simulink model "AOO"  (R2022a)
settings: Solver=FixedStepAuto  StartTime=0.0  StopTime=inf  FixedStep=1e-3  RelTol=1e-3  EnableMultiTasking=on
undefined symbols (not defined in the file): D10, D11, D12, D2, D4, D5, D7, D8, D9, PTA0, PTA2, PTB23, PTB9, PTC3, PTC4, PTD0, PTD2, PTD3
libraries: frdmk64flib x9
settings Model: ExtModeTrigDuration=5  Creator=ethan  LastModifiedBy=taimu
settings OptimizationCC: EnhancedBackFolding=on  PassReuseOutputArgsAs=Individual arguments  ZeroExternalMemoryAtStartup=off  ZeroInternalMemoryAtStartup=off  MaxStackSize=64  OptimizeBlockOrder=speed  DifferentSizesBufferReuse=on  OptimizationCustomize=off  EfficientTunableParamExpr=on
settings DebuggingCC: ParameterTunabilityLossMsg=error
settings HardwareCC: ProdBitPerPointer=32  ProdBitPerSizeT=32  ProdBitPerPtrDiffT=32  ProdLargestAtomicInteger=Long  ProdLargestAtomicFloat=Double  ProdWordSize=32  ProdHWDeviceType=ARM Compatible->ARM Cortex
settings SFSimCC: MATLABDynamicMemAlloc=off
settings RTWCC: SystemTargetFile=ert.tlc  HardwareBoard=NXP FRDM-K64F  TLCOptions="-aInlineSetEventsForThisBaseRateFcn=TLC_FALSE -aSuppressMultiTaskScheduler=TLC_FALSE  -aRateBasedStepFcn=0"  TemplateMakefile=ert_default_tmf  Toolchain=GNU Tools for ARM Embedded Processors
settings CodeAppCC: ForceParamTrailComments=on  IgnoreCustomStorageClasses=off  OperatorAnnotations=on  SimulinkDataObjDesc=on  SFDataObjDesc=on  InsertBlockDesc=on
settings ERTTargetCC: ExtModeTransport=4  ExtModeMexFile=sendToCommService

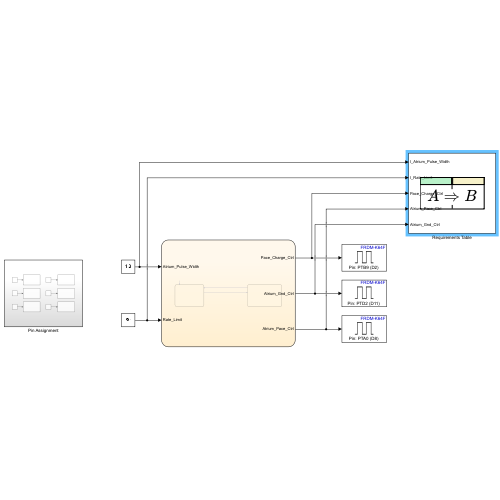
[thumbnail: Simulink's stored preview of the top-level diagram]
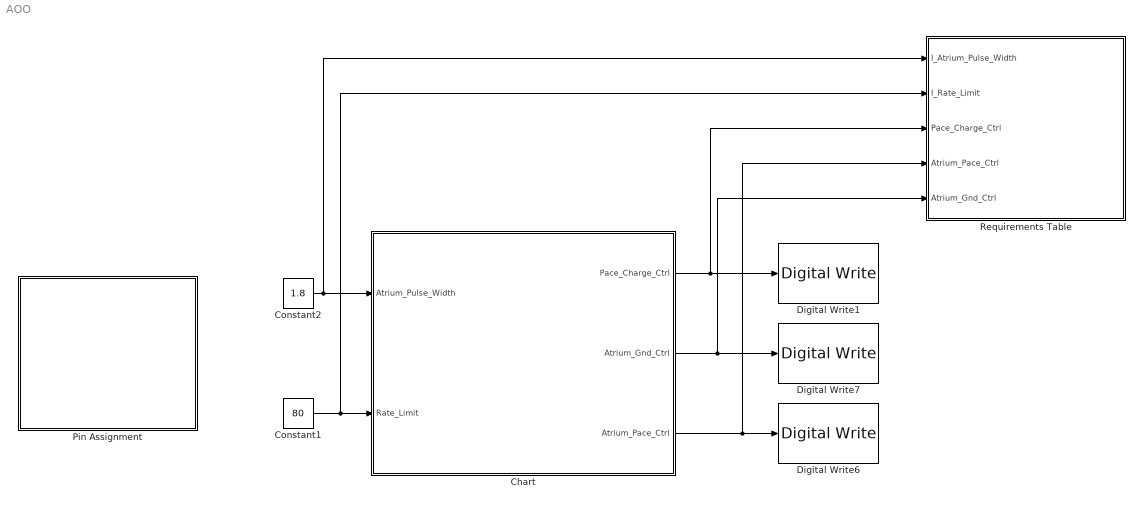
== system AOO ==
  Chart : Stateflow chart  TreatAsAtomicUnit=on
  Constant1 : Constant  Value=80  OutDataTypeStr=double
  Constant2 : Constant  Value=1.8
  Digital Write1 : frdmk64flib/Digital Write  Whichpin=PTB9 (D2)
  Digital Write6 : frdmk64flib/Digital Write  Whichpin=PTA0 (D8)
  Digital Write7 : frdmk64flib/Digital Write  Whichpin=PTD2 (D11)
  Pin Assignment : Subsystem
  Requirements Table : Requirements Table  TreatAsAtomicUnit=on
  wires:
  Chart/1(Pace_Charge_Ctrl) -> Requirements Table/3(Pace_Charge_Ctrl), Digital Write1/1
  Constant1/1 -> Requirements Table/2(I_Rate_Limit), Chart/2(Rate_Limit)
  Constant2/1 -> Requirements Table/1(I_Atrium_Pulse_Width), Chart/1(Atrium_Pulse_Width)
  Chart/2(Atrium_Gnd_Ctrl) -> Requirements Table/5(Atrium_Gnd_Ctrl), Digital Write7/1
  Chart/3(Atrium_Pace_Ctrl) -> Requirements Table/4(Atrium_Pace_Ctrl), Digital Write6/1

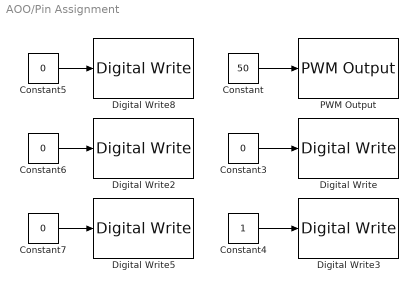
== system AOO/Pin Assignment ==
  Constant : Constant  Value=50  OutDataTypeStr=int8
  Constant{3,5..7} (4 alike) : Constant  Value=0  OutDataTypeStr=int8
  Constant4 : Constant  OutDataTypeStr=int8
  Digital Write : frdmk64flib/Digital Write  Whichpin=PTD3 (D12)
  Digital Write2 : frdmk64flib/Digital Write  Whichpin=PTC4 (D9)
  Digital Write3 : frdmk64flib/Digital Write  Whichpin=PTD0 (D10)
  Digital Write5 : frdmk64flib/Digital Write  Whichpin=PTC3 (D7)
  Digital Write8 : frdmk64flib/Digital Write  Whichpin=PTB23 (D4)
  PWM Output : frdmk64flib/PWM Output  Whichpin=PTA2 (D5)  InitialFrequency=2000  InitialDutyCycle=0
  wires:
  Constant4/1 -> Digital Write3/1
  Constant/1 -> PWM Output/1
  Constant7/1 -> Digital Write5/1
  Constant5/1 -> Digital Write8/1
  Constant6/1 -> Digital Write2/1
  Constant3/1 -> Digital Write/1

== stateflow chart AOO/Requirements Table ==
  (default) -> (junction 1073741860)
  (junction 1073741860) -> (junction 1073741861) : {
      | % SF_REQ_REV_07
      | }
  (junction 1073741861) -> (junction 1073741863) : {
      | % HEADER_ASSIGNMENTS
      |
      | }
  (junction 1073741863) -> (junction 1073741865) : {
      | % START_A_4
      | }
  (junction 1073741865) -> (junction 1073741867) : {
      | }
  (junction 1073741867) -> (junction 1073741869)
  (junction 1073741869) -> (junction 1073741871) : {
      | }
  (junction 1073741871) -> (junction 1073741873) : {
      | % END_A_4
      | }
  (junction 1073741873) -> (junction 1073741915) : {
      | % START_R_1
      | }
  (junction 1073741915) -> (junction 1073741917) : {
      | }
  (junction 1073741917) -> (junction 1073741919)
  (junction 1073741919) -> (junction 1073741921) [order 1] : [(((I_Rate_Limit) == (30)) || ((I_Rate_Limit) == (35)) || ((I_Rate_Limit) == (40)) || ((I_Rate_Limit) == (45)) || ((I_Rate_Limit) == (50)) || ((I_Rate_Limit) == (51)) || ((I_Rate_Limit) == (52)) || ((I_Rate_Limit) == (53)) || ((I_Rate_Limit) == (54)) || ((I_Rate_Limit) == (55)) || ((I_Rate_Limit) == (56)) || ((I_Rate_Limit) == (57)) || ((I_Rate_Limit) == (58)) || ((I_Rate_Limit) == (59)) || ((I_Rate_Limit) == (60)) || ((I_Rate_Limit) == (61)) || ((I_Rate_Limit) == (62)) || ((I_Rate_Limit) == (63)) || ((I_Rate_Limit) == (64)) || ((I_Rate_Limit) == (65)) || ((I_Rate_Limit) == (66)) || ((I_Rate_Limit) == (67)) || ((I_Rate_Limit) == (68)) || ((I_Rate_Limit) == (69)) || ((I_Rate_Limit) == (70)) || ((I_Rate_Limit) == (71)) || ((I_Rate_Limit) == (72)) || ((I_Rate_Limit) == (73)) || ((I_Rate_Limit) == (74)) || ((I_Rate_Limit) == (75)) || ((I_Rate_Limit) == (76)) || ((I_Rate_Limit) == (77)) || ((I_Rate_Limit) == (78)) || ((I_Rate_Limit) == (79)) || ((I_Rate_Limit) == (80)) || ((I_Rate_Limit) == (81)) || ((I_Rate_Limit) == (82)) || ((I_Rate_Limit) == (83)) || ((I_Rate_Limit) == (84)) || ((I_Rate_Limit) == (85)) || ((I_Rate_Limit) == (86)) || ((I_Rate_Limit) == (87)) || ((I_Rate_Limit) == (88)) || ((I_Rate_Limit) == (89)) || ((I_Rate_Limit) == (90)) || ((I_Rate_Limit) == (95)) || ((I_Rate_Limit) == (100)) || ((I_Rate_Limit) == (105)) || ((I_Rate_Limit) == (110)) || ((I_Rate_Limit) == (115)) || ((I_Rate_Limit) == (120)) || ((I_Rate_Limit) == (125)) || ((I_Rate_Limit) == (130)) || ((I_Rate_Limit) == (135)) || ((I_Rate_Limit) == (140)) || ((I_Rate_Limit) == (145)) || ((I_Rate_Limit) == (150)) || ((I_Rate_Limit) == (155)) || ((I_Rate_Limit) == (160)) || ((I_Rate_Limit) == (165)) || ((I_Rate_Limit) == (170)) || ((I_Rate_Limit) == (175))) && (((I_Atrium_Pulse_Width) == (0.05)) || ((I_Atrium_Pulse_Width) == (0.1)) || ((I_Atrium_Pulse_Width) == (0.2)) || ((I_Atrium_Pulse_Width) == (0.3)) || ((I_Atrium_Pulse_Width) == (0.4)) || ((I_Atrium_Pulse_Width) == (0.5)) || ((I_Atrium_Pulse_Width) == (0.6)) || ((I_Atrium_Pulse_Width) == (0.7)) || ((I_Atrium_Pulse_Width) == (0.8)) || ((I_Atrium_Pulse_Width) == (0.9)) || ((I_Atrium_Pulse_Width) == (1)) || ((I_Atrium_Pulse_Width) == (1.1)) || ((I_Atrium_Pulse_Width) == (1.2)) || ((I_Atrium_Pulse_Width) == (1.3)) || ((I_Atrium_Pulse_Width) == (1.4)) || ((I_Atrium_Pulse_Width) == (1.5)) || ((I_Atrium_Pulse_Width) == (1.6)) || ((I_Atrium_Pulse_Width) == (1.7)) || ((I_Atrium_Pulse_Width) == (1.8)) || ((I_Atrium_Pulse_Width) == (1.9)))]
  (junction 1073741919) -> (junction 1073741927) [order 2]
  (junction 1073741921) -> (junction 1073741923) : {
      | reqtable_postcondition(((Pace_Charge_Ctrl == true && Atrium_Gnd_Ctrl == true && Atrium_Pace_Ctrl == false) || (Pace_Charge_Ctrl == false && Atrium_Gnd_Ctrl == false && Atrium_Pace_Ctrl == true)), 'R:1');
      |
      |
      | }
  (junction 1073741923) -> (junction 1073741925) : {
      | }
  (junction 1073741925) -> (junction 1073741927)
  (junction 1073741927) -> (junction 1073741929)
  (junction 1073741929) -> (junction 1073741931) : {
      | % END_R_1
      | }
  data: I_Atrium_Pulse_Width input; I_Rate_Limit input; Pace_Charge_Ctrl input; Atrium_Pace_Ctrl input; Atrium_Gnd_Ctrl input

== stateflow chart AOO/Chart ==
  state Charge_C22
    entry:
    Atrium_Pace_Ctrl = false;
    Atrium_Gnd_Ctrl = true;
    Pace_Charge_Ctrl = true;
  state Discharge_C22
    entry:
    Pace_Charge_Ctrl = false;
    Atrium_Pace_Ctrl = true;
    Atrium_Gnd_Ctrl = false;
  (default) -> Charge_C22
  Discharge_C22 -> Charge_C22 : after(Atrium_Pulse_Width,msec)
  Charge_C22 -> Discharge_C22 : after((60000/Rate_Limit)-Atrium_Pulse_Width,msec)
  data: Pace_Charge_Ctrl output; Atrium_Gnd_Ctrl output; Atrium_Pace_Ctrl output; Atrium_Pulse_Width input; Rate_Limit input
